simulink model "sub1"  (R2015a)
settings: Solver=ode45  StartTime=0.0  StopTime=10.0  RelTol=1e-3
settings Model: Creator=Frank  LastModifiedBy=Frank

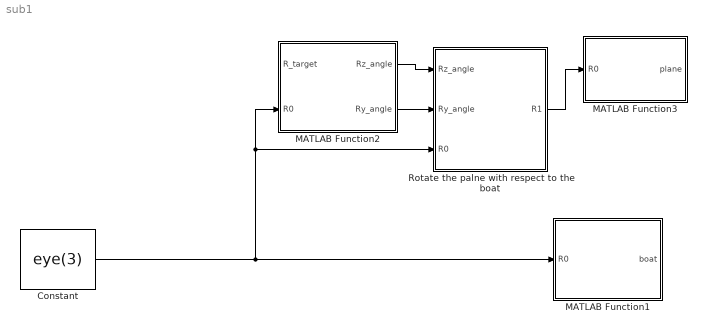
== system sub1 ==
  Constant : Constant  Value=eye(3)  VectorParams1D=off
  MATLAB Function1 : MATLAB Function  TreatAsAtomicUnit=on
  MATLAB Function2 : MATLAB Function  TreatAsAtomicUnit=on
  MATLAB Function3 : MATLAB Function  TreatAsAtomicUnit=on
  "Rotate the palne with respect to the boat " : MATLAB Function  TreatAsAtomicUnit=on
  wires:
  MATLAB Function2/1(Rz_angle) -> "Rotate the palne with respect to the boat "/1(Rz_angle)
  MATLAB Function2/2(Ry_angle) -> "Rotate the palne with respect to the boat "/2(Ry_angle)
  "Rotate the palne with respect to the boat "/1(R1) -> MATLAB Function3/1(R0)
  Constant/1 -> "Rotate the palne with respect to the boat "/3(R0), MATLAB Function2/2(R0), MATLAB Function1/1(R0)

== matlab function sub1/MATLAB Function2 ==
  data: R_target input; Rz_angle output; R0 input; Ry_angle output
function [Rz_angle,Ry_angle] = fcn(R_target,R0)
%#codegen

y = u;

== matlab function sub1/MATLAB Function1 ==
  data: R0 input; boat output
function boat = get_boat(R0)
%#codegen

y = u;

== matlab function sub1/Rotate the palne with respect to the boat  ==
  data: Rz_angle input; R1 output; Ry_angle input; R0 input
function R1 = rotate_plane(Rz_angle,Ry_angle,R0)
%#codegen
Rz
y = u;

== matlab function sub1/MATLAB Function3 ==
  data: R0 input; plane output
function plane = get_plane(R0)
%#codegen

y = u;
